simulink model "SMC_ThreeLayerApproach5TrackingNew"  (R2019b)
settings: Solver=FixedStepAuto  StartTime=0.0  StopTime=10.0  FixedStep=0.002  RelTol=1e-3
libraries: robotcorelib x1
settings Model: Creator=USER  LastModifiedBy=USER

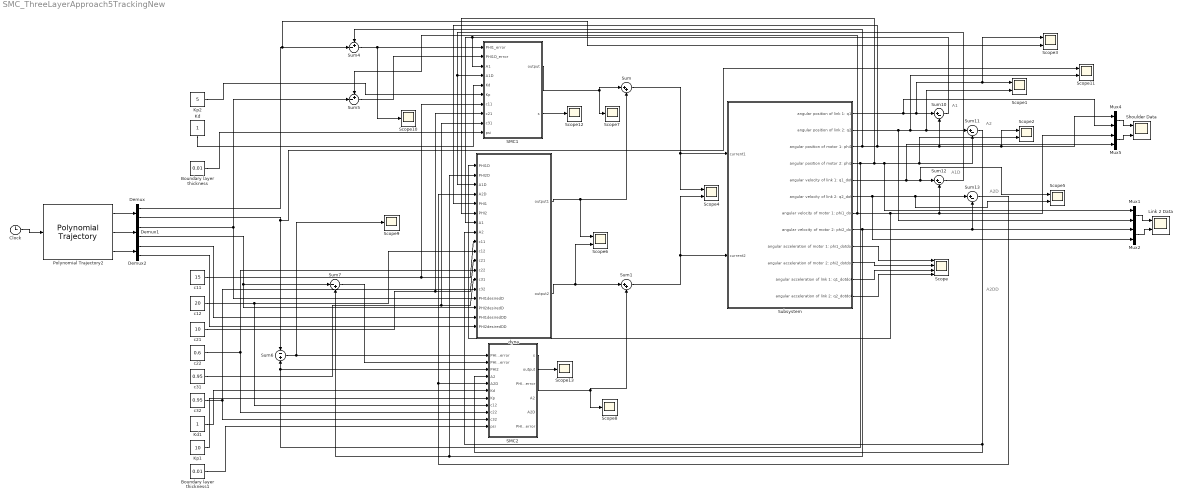
== system SMC_ThreeLayerApproach5TrackingNew ==
  note: A2D
  note: A2
  note: A1
  note: A1D
  note: A2DD
  Boundary layer thickness : Constant  Value=0.01
  Boundary layer thickness1 : Constant  Value=0.01  VectorParams1D=off
  Clock : Clock
  Demux : Demux  Outputs=2
  Demux1 : Demux  Outputs=2
  Demux2 : Demux  Outputs=2
  Kd : Constant
  Kd1 : Constant
  Kp1 : Constant  Value=10
  Kp2 : Constant  Value=5
  Link 2 Data : Scope  NumInputPorts=2
  Mux{1..2,4..5} (4 alike) : Mux  Inputs=2
  Polynomial Trajectory2 : robotcorelib/Polynomial Trajectory  WaypointSource=Internal  Waypoints=[ 0, pi/2; 0, pi/4 ]  TimePoints=[0,5]  TimeInterval=[ 1, 4 ]  Method=Cubic Polynomial  ParameterSource=Internal  VelocityBoundaryCondition=zeros( 2, 2 )  AccelerationBoundaryCondition=zeros( 2, 5 )  SimulateUsing=Interpreted execution
      settings: SourceProductName=Robotics System Toolbox  SourceProductBaseCode=RO
  SMC1 : MATLAB Function  TreatAsAtomicUnit=on
  SMC2 : MATLAB Function  TreatAsAtomicUnit=on
  Scope : Scope  NumInputPorts=4
  Scope{1..6,11} (7 alike) : Scope  NumInputPorts=2
  Scope{7..10,12..13} (6 alike) : Scope
  Shoulder Data : Scope  NumInputPorts=2
  Subsystem : Subsystem
  Sum : Sum  Inputs=|++
  Sum1 : Sum  Inputs=|++
  Sum{10..13} (4 alike) : Sum  Inputs=|+-
  Sum4 : Sum  Inputs=+-|
  Sum5 : Sum  Inputs=+-|
  Sum6 : Sum  Inputs=-|+
  Sum7 : Sum  Inputs=|-+
  c11 : Constant  Value=15
  c12 : Constant  Value=20
  c21 : Constant  Value=10
  c22 : Constant  Value=0.6
  c31 : Constant  Value=0.95
  c32 : Constant  Value=0.95
  dyna : MATLAB Function  TreatAsAtomicUnit=on
  wires:
  Mux2/1 -> Link 2 Data/2
  Kp1/1 -> SMC2/7(Kp)
  Sum7/1 -> SMC2/2("PHI2D_error ")
  Subsystem/12(angular acceleration of link 2: q2_dotdot) -> Scope/4
  Demux1/2 -> dyna/16(PHI2desiredD), Sum7/1
  Sum/1 -> Scope4/1, Subsystem/1(current1)
  Subsystem/10(angular acceleration of motor 2: phi2_dotdot) -> Scope/2
  Sum5/1 -> SMC1/2(PHI1D_error)
  c32/1 -> SMC2/10(c32), dyna/14(c32)
  Subsystem/9(angular acceleration of motor 1: phi1_dotdot) -> Scope/1
  Subsystem/8(angular velocity of motor 2: phi2_dot) -> dyna/2(PHI2D), Sum7/2, Mux2/1, Sum13/2
  dyna/1(output1) -> Scope6/1, Sum/2
  Subsystem/11(angular acceleration of link 1: q1_dotdot) -> Scope/3
  SMC1/1(output) -> Sum/1, Scope7/1
  c21/1 -> SMC1/8(c21), dyna/11(c21)
  Subsystem/6(angular velocity of link 2: q2_dot) -> Mux2/2, Scope5/2, Sum13/1
  Sum10/1 -> dyna/7(A1), SMC1/3(A1)
  Subsystem/4(angular position of motor 2: phi2) -> dyna/6(PHI2), Mux1/1, Scope2/2, Sum11/2, SMC2/3(PHI2), Sum6/2
  c31/1 -> SMC1/9(c31), dyna/13(c31)
  Sum12/1 -> SMC1/4(A1D), dyna/3(A1D)
  Sum11/1 -> SMC2/4("A2 "), dyna/8(A2)
  Kd/1 -> SMC1/5(Kd)
  Subsystem/2(angular position of link 2: q2) -> Mux1/2, Scope11/2, Scope1/2, Sum11/1
  Kd1/1 -> SMC2/6(Kd)
  Boundary layer thickness1/1 -> SMC2/11(psi)
  SMC2/2(output) -> Sum1/2, Scope8/1
  Subsystem/5(angular velocity of link 1: q1_dot) -> Mux5/2, Scope5/1, Sum12/1
  c11/1 -> SMC1/7(c11), dyna/9(c11)
  Sum4/1 -> Scope10/1, SMC1/1(PHI1_error)
  Subsystem/1(angular position of link 1: q1) -> Mux4/2, Scope3/1, Scope1/1, Sum10/1
  Mux4/1 -> Shoulder Data/1
  dyna/2(output2) -> Scope6/2, Sum1/1
  Sum6/1 -> Scope9/1, SMC2/1("PHI2_error ")
  Subsystem/7(angular velocity of motor 1: phi1_dot) -> dyna/1(PHI1D), Mux5/1, Sum12/2, Sum5/1
  Mux5/1 -> Shoulder Data/2
  Subsystem/3(angular position of motor 1: phi1) -> dyna/5(PHI1), Mux4/1, Scope2/1, Sum10/2, Sum4/1
  Sum13/1 -> dyna/4(A2D), SMC2/5("A2D ")
  Demux/2 -> Scope11/1, Sum6/1
  Sum1/1 -> Subsystem/2("current2 "), Scope4/2
  Demux/1 -> Scope3/2, Sum4/2
  Mux1/1 -> Link 2 Data/1
  c22/1 -> SMC2/9(c22), dyna/12(c22)
  Boundary layer thickness/1 -> SMC1/10(psi)
  Clock/1 -> Polynomial Trajectory2/1
  Kp2/1 -> SMC1/6(Kp)
  c12/1 -> SMC2/8(c12), dyna/10(c12)
  Polynomial Trajectory2/1 -> Demux/1
  Polynomial Trajectory2/2 -> Demux1/1
  Polynomial Trajectory2/3 -> Demux2/1
  Demux1/1 -> Sum5/2, dyna/15(PHI1desiredD)
  Demux2/1 -> dyna/17(PHI1desiredDD)
  Demux2/2 -> dyna/18(PHI2desiredDD)
  SMC1/2(s) -> Scope12/1
  SMC2/1(s) -> Scope13/1

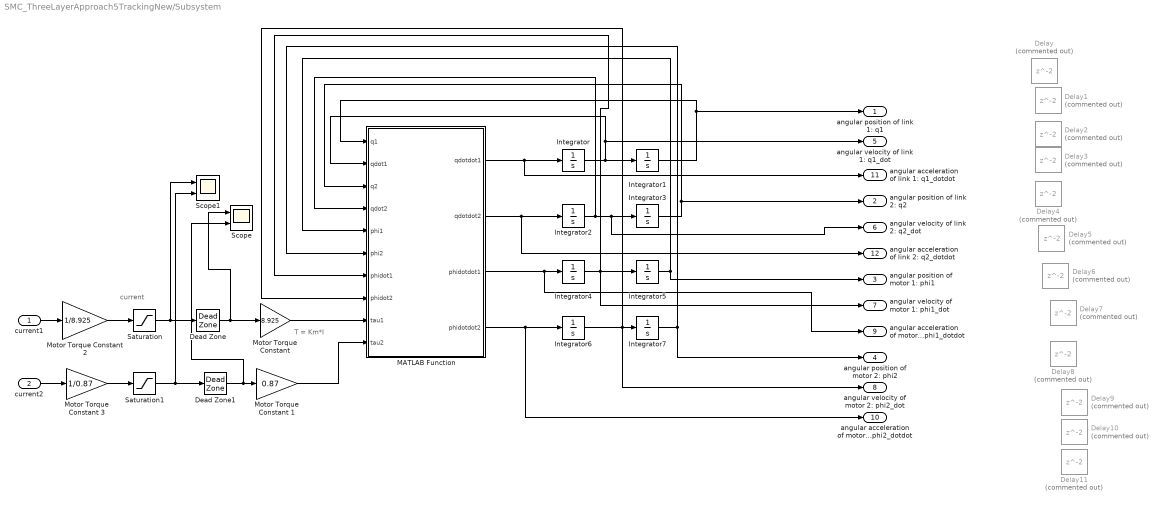
== system SMC_ThreeLayerApproach5TrackingNew/Subsystem ==
  note: current
  note: T = Km*I
  current1 : Inport
  "current2 " : Inport  Port=2
  Dead Zone : DeadZone  LowerValue=-0.165  UpperValue=0.183  ZeroCross=off  SaturateOnIntegerOverflow=on
  Dead Zone1 : DeadZone  LowerValue=-0.165  UpperValue=0.183  ZeroCross=off  SaturateOnIntegerOverflow=on
  Delay{,1..11} (12 alike) : Delay  Commented=on  SampleTime=0.002
  Integrator{,1..7} (8 alike) : Integrator
  MATLAB Function : MATLAB Function  TreatAsAtomicUnit=on
  "Motor Torque Constant " : Gain  Gain=8.925
  Motor Torque Constant 1 : Gain  Gain=0.87
  Motor Torque Constant 2 : Gain  Gain=1/8.925
  Motor Torque Constant 3 : Gain  Gain=1/0.87
  Saturation : Saturate  UpperLimit=0.94  LowerLimit=-0.94  ZeroCross=off
  Saturation1 : Saturate  UpperLimit=0.94  LowerLimit=-0.94  ZeroCross=off
  Scope : Scope  NumInputPorts=2
  Scope1 : Scope  NumInputPorts=2
  angular position of link 1: q1 : Outport
  angular position of link 2: q2 : Outport  Port=2
  angular position of motor 1: phi1 : Outport  Port=3
  angular position of motor 2: phi2 : Outport  Port=4
  angular velocity of link 1: q1_dot : Outport  Port=5
  angular velocity of link 2: q2_dot : Outport  Port=6
  angular velocity of motor 1: phi1_dot : Outport  Port=7
  angular velocity of motor 2: phi2_dot : Outport  Port=8
  angular acceleration of motor 1: phi1_dotdot : Outport  Port=9
  angular acceleration of motor 2: phi2_dotdot : Outport  Port=10
  angular acceleration of link 1: q1_dotdot : Outport  Port=11
  angular acceleration of link 2: q2_dotdot : Outport  Port=12
  wires:
  Saturation/1 -> Scope1/1, Dead Zone/1
  "Motor Torque Constant "/1 -> MATLAB Function/9(tau1)
  Motor Torque Constant 1/1 -> MATLAB Function/10(tau2)
  Dead Zone/1 -> Scope/1, "Motor Torque Constant "/1
  Dead Zone1/1 -> Scope/2, Motor Torque Constant 1/1
  current1/1 -> Motor Torque Constant 2/1
  "current2 "/1 -> Motor Torque Constant 3/1
  Motor Torque Constant 2/1 -> Saturation/1
  Motor Torque Constant 3/1 -> Saturation1/1
  Saturation1/1 -> Scope1/2, Dead Zone1/1
  Integrator1/1 -> angular position of link 1: q1/1, MATLAB Function/1(q1)
  Integrator/1 -> angular velocity of link 1: q1_dot/1, MATLAB Function/2(qdot1), Integrator1/1
  MATLAB Function/1(qdotdot1) -> angular acceleration of link 1: q1_dotdot/1, Integrator/1
  Integrator3/1 -> angular position of link 2: q2/1, MATLAB Function/3(q2)
  Integrator2/1 -> angular velocity of link 2: q2_dot/1, Integrator3/1, MATLAB Function/4(qdot2)
  MATLAB Function/2(qdotdot2) -> angular acceleration of link 2: q2_dotdot/1, Integrator2/1
  Integrator5/1 -> angular position of motor 1: phi1/1, MATLAB Function/5(phi1)
  MATLAB Function/3(phidotdot1) -> angular acceleration of motor 1: phi1_dotdot/1, Integrator4/1
  Integrator4/1 -> angular velocity of motor 1: phi1_dot/1, Integrator5/1, MATLAB Function/7(phidot1)
  Integrator6/1 -> angular velocity of motor 2: phi2_dot/1, MATLAB Function/8(phidot2), Integrator7/1
  MATLAB Function/4(phidotdot2) -> angular acceleration of motor 2: phi2_dotdot/1, Integrator6/1
  Integrator7/1 -> angular position of motor 2: phi2/1, MATLAB Function/6(phi2)

== matlab function SMC_ThreeLayerApproach5TrackingNew/dyna ==
  data: output1 output; PHI1D input; PHI2D input; A1D input; A2D input; output2 output; PHI1 input; PHI2 input; A1 input; A2 input; c11 input; c12 input; c21 input; c22 input; c31 input; c32 input; PHI1desiredD input; PHI2desiredD input; PHI1desiredDD input; PHI2desiredDD input
function [output1, output2]= dyna(PHI1D, PHI2D,A1D, A2D, PHI1, PHI2, A1, A2, c11, c12, c21, c22, c31, c32, PHI1desiredD, PHI2desiredD,PHI1desiredDD,PHI2desiredDD)
%Electrical School values
L1 = 0.343;
L2 = 0.267;
Lc1 = 0.1590;
Lc2 = 0.0550;
m1 = 1.51;
m2 = 0.87326;
I1 = 0.0392;
I2 = 0.0081;
B1 = 0.070364;
B2 = 0.028211;
Bm1 =4.5;
Bm2 = 0.5;
Ks1 = 9;
Ks2 = 4;
Ir1 = 0.0628;
Ir2 = 0.0026;
    
A1desiredD = 0;
A2desiredD = 0;
% PHI1desiredD = 0;
% PHI2desiredD = 0;
A1desiredDD = 0;
A2desiredDD = 0;
% PHI1desiredDD = 0;
% PHI2desiredDD = 0;

%derived from SMC_threeLayer.mlx
output1 = (c21*(A1D - A1desiredD) - PHI1desiredDD + c11*(PHI1D - PHI1desiredD) - c31*(A1desiredDD - (2*A2*I2^2*Ir1*Ks2 - 2*A1*I1^2*I2*Ks1 - 2*A1*I2^2*Ir1*Ks1 - 2*A1*I1*I2^2*Ks1 - A1*Ks1*L1^2*Lc2^4*m2^3 - A1*Ks1*L1^4*Lc2^2*m2^3 - 2*A1*I2^2*Ks1*L1^2*m2 - 2*A1*I2*Ks1*L1^4*m2^2 - 2*A1*I2^2*Ks1*Lc1^2*m1 - 2*A1*I1^2*Ks1*Lc2^2*m2 - 2*A1*I2*Ks1*Lc1^4*m1^2 - 2*A1*I1*Ks1*Lc2^4*m2^2 - 2*A1*Ir1*Ks1*Lc2^4*m2^2 + 2*A2*Ir1*Ks2*Lc2^4*m2^2 - 2*A1*I1*I2*Ir1*Ks1 + 2*A2*I1*I2*Ir1*Ks2 + A1*Ks1*L1^2*Lc2^4*m2^3*cos(2*A2 + 2*PHI2) + A1*Ks1*L1^4*Lc2^2*m2^3*cos(2*A2 + 2*PHI2) + A1*Ks1*L1^3*Lc2^3*m2^3*cos(3*A2 + 3*PHI2) - 3*A1*I1*Ks1*L1^2*Lc2^2*m2^2 - 3*A1*I2*Ks1*L1^2*Lc2^2*m2^2 - 2*A1*Ir1*Ks1*L1^2*Lc2^2*m2^2 + 4*A2*Ir1*Ks2*L1^2*Lc2^2*m2^2 - A1*Ks1*L1^3*Lc2^3*m2^3*cos(A2 + PHI2) + 2*A1D^2*Ir1*L1*Lc2^5*m2^3*sin(A2 + PHI2) + 2*A2D^2*Ir1*L1*Lc2^5*m2^3*sin(A2 + PHI2) - 2*A1*Ks1*Lc1^2*Lc2^4*m1*m2^2 - 2*A1*Ks1*Lc1^4*Lc2^2*m1^2*m2 + 2*Ir1*L1*Lc2^5*PHI1D^2*m2^3*sin(A2 + PHI2) + 2*Ir1*L1*Lc2^5*PHI2D^2*m2^3*sin(A2 + PHI2) + 3*A1D^2*Ir1*L1^2*Lc2^4*m2^3*sin(2*A2 + 2*PHI2) + A1D^2*Ir1*L1^4*Lc2^2*m2^3*sin(2*A2 + 2*PHI2) + 2*A2D^2*Ir1*L1^2*Lc2^4*m2^3*sin(2*A2 + 2*PHI2) + A1D^2*Ir1*L1^3*Lc2^3*m2^3*sin(3*A2 + 3*PHI2) - 4*A1*I1*I2*Ks1*L1^2*m2 - 4*A1*I1*I2*Ks1*Lc1^2*m1 - 4*A1*I1*I2*Ks1*Lc2^2*m2 - 2*A1*I2*Ir1*Ks1*L1^2*m2 + 2*A2*I2*Ir1*Ks2*L1^2*m2 - 2*A1*I2*Ir1*Ks1*Lc1^2*m1 - 2*A1*I1*Ir1*Ks1*Lc2^2*m2 - 4*A1*I2*Ir1*Ks1*Lc2^2*m2 + 2*A2*I2*Ir1*Ks2*Lc1^2*m1 + 2*A2*I1*Ir1*Ks2*Lc2^2*m2 + 4*A2*I2*Ir1*Ks2*Lc2^2*m2 + 3*Ir1*L1^2*Lc2^4*PHI1D^2*m2^3*sin(2*A2 + 2*PHI2) + Ir1*L1^4*Lc2^2*PHI1D^2*m2^3*sin(2*A2 + 2*PHI2) + 2*Ir1*L1^2*Lc2^4*PHI2D^2*m2^3*sin(2*A2 + 2*PHI2) + Ir1*L1^3*Lc2^3*PHI1D^2*m2^3*sin(3*A2 + 3*PHI2) + 3*A1D^2*Ir1*L1^3*Lc2^3*m2^3*sin(A2 + PHI2) + 2*A2D^2*Ir1*L1^3*Lc2^3*m2^3*sin(A2 + PHI2) + 3*Ir1*L1^3*Lc2^3*PHI1D^2*m2^3*sin(A2 + PHI2) + 2*Ir1*L1^3*Lc2^3*PHI2D^2*m2^3*sin(A2 + PHI2) - 3*A1*Ks1*L1^2*Lc1^2*Lc2^2*m1*m2^2 - 4*A1*I1*Ks1*L1*Lc2^3*m2^2*cos(A2 + PHI2) - 4*A1*I2*Ks1*L1^3*Lc2*m2^2*cos(A2 + PHI2) - 4*A1*Ir1*Ks1*L1*Lc2^3*m2^2*cos(A2 + PHI2) + 6*A2*Ir1*Ks2*L1*Lc2^3*m2^2*cos(A2 + PHI2) + 2*A2*Ir1*Ks2*L1^3*Lc2*m2^2*cos(A2 + PHI2) + 4*A1D*A2D*Ir1*L1*Lc2^5*m2^3*sin(A2 + PHI2) + 2*A1D^2*I2^2*Ir1*L1*Lc2*m2*sin(A2 + PHI2) + 2*A2D^2*I2^2*Ir1*L1*Lc2*m2*sin(A2 + PHI2) + 4*A1D*Ir1*L1*Lc2^5*PHI1D*m2^3*sin(A2 + PHI2) + 4*A1D*Ir1*L1*Lc2^5*PHI2D*m2^3*sin(A2 + PHI2) + 4*A2D*Ir1*L1*Lc2^5*PHI1D*m2^3*sin(A2 + PHI2) + 4*A2D*Ir1*L1*Lc2^5*PHI2D*m2^3*sin(A2 + PHI2) - 4*A1*I2*Ks1*L1^2*Lc1^2*m1*m2 - 4*A1*I1*Ks1*Lc1^2*Lc2^2*m1*m2 - 4*A1*I2*Ks1*Lc1^2*Lc2^2*m1*m2 - 2*A1*Ir1*Ks1*Lc1^2*Lc2^2*m1*m2 + 2*A2*Ir1*Ks2*Lc1^2*Lc2^2*m1*m2 + 2*I2^2*Ir1*L1*Lc2*PHI1D^2*m2*sin(A2 + PHI2) + 2*I2^2*Ir1*L1*Lc2*PHI2D^2*m2*sin(A2 + PHI2) + A1*I1*Ks1*L1^2*Lc2^2*m2^2*cos(2*A2 + 2*PHI2) + A1*I2*Ks1*L1^2*Lc2^2*m2^2*cos(2*A2 + 2*PHI2) + 2*A2*Ir1*Ks2*L1^2*Lc2^2*m2^2*cos(2*A2 + 2*PHI2) + 4*A1D*A2D*Ir1*L1^2*Lc2^4*m2^3*sin(2*A2 + 2*PHI2) + 4*Ir1*L1*Lc2^5*PHI1D*PHI2D*m2^3*sin(A2 + PHI2) + 6*A1D*Ir1*L1^2*Lc2^4*PHI1D*m2^3*sin(2*A2 + 2*PHI2) + 2*A1D*Ir1*L1^4*Lc2^2*PHI1D*m2^3*sin(2*A2 + 2*PHI2) + 4*A1D*Ir1*L1^2*Lc2^4*PHI2D*m2^3*sin(2*A2 + 2*PHI2) + 4*A2D*Ir1*L1^2*Lc2^4*PHI1D*m2^3*sin(2*A2 + 2*PHI2) + 2*A1D*Ir1*L1^3*Lc2^3*PHI1D*m2^3*sin(3*A2 + 3*PHI2) + 4*A2D*Ir1*L1^2*Lc2^4*PHI2D*m2^3*sin(2*A2 + 2*PHI2) + 4*Ir1*L1^2*Lc2^4*PHI1D*PHI2D*m2^3*sin(2*A2 + 2*PHI2) + 4*A1D*A2D*Ir1*L1^3*Lc2^3*m2^3*sin(A2 + PHI2) + 2*A1D^2*I1*Ir1*L1*Lc2^3*m2^2*sin(A2 + PHI2) + 4*A1D^2*I2*Ir1*L1*Lc2^3*m2^2*sin(A2 + PHI2) + 2*A1D^2*I2*Ir1*L1^3*Lc2*m2^2*sin(A2 + PHI2) + 2*A2D^2*I1*Ir1*L1*Lc2^3*m2^2*sin(A2 + PHI2) + 4*A2D^2*I2*Ir1*L1*Lc2^3*m2^2*sin(A2 + PHI2) + 2*A2D^2*I2*Ir1*L1^3*Lc2*m2^2*sin(A2 + PHI2) + 6*A1D*Ir1*L1^3*Lc2^3*PHI1D*m2^3*sin(A2 + PHI2) + 4*A1D*Ir1*L1^3*Lc2^3*PHI2D*m2^3*sin(A2 + PHI2) + 4*A2D*Ir1*L1^3*Lc2^3*PHI1D*m2^3*sin(A2 + PHI2) + 4*A2D*Ir1*L1^3*Lc2^3*PHI2D*m2^3*sin(A2 + PHI2) + 2*I1*Ir1*L1*Lc2^3*PHI1D^2*m2^2*sin(A2 + PHI2) + 2*I1*Ir1*L1*Lc2^3*PHI2D^2*m2^2*sin(A2 + PHI2) + 4*I2*Ir1*L1*Lc2^3*PHI1D^2*m2^2*sin(A2 + PHI2) + 2*I2*Ir1*L1^3*Lc2*PHI1D^2*m2^2*sin(A2 + PHI2) + 4*I2*Ir1*L1*Lc2^3*PHI2D^2*m2^2*sin(A2 + PHI2) + 2*I2*Ir1*L1^3*Lc2*PHI2D^2*m2^2*sin(A2 + PHI2) + 4*Ir1*L1^3*Lc2^3*PHI1D*PHI2D*m2^3*sin(A2 + PHI2) + A1D^2*I1*Ir1*L1^2*Lc2^2*m2^2*sin(2*A2 + 2*PHI2) + 3*A1D^2*I2*Ir1*L1^2*Lc2^2*m2^2*sin(2*A2 + 2*PHI2) + 2*A2D^2*I2*Ir1*L1^2*Lc2^2*m2^2*sin(2*A2 + 2*PHI2) + I1*Ir1*L1^2*Lc2^2*PHI1D^2*m2^2*sin(2*A2 + 2*PHI2) + 3*I2*Ir1*L1^2*Lc2^2*PHI1D^2*m2^2*sin(2*A2 + 2*PHI2) + 2*I2*Ir1*L1^2*Lc2^2*PHI2D^2*m2^2*sin(2*A2 + 2*PHI2) - 4*A1*Ks1*L1*Lc1^2*Lc2^3*m1*m2^2*cos(A2 + PHI2) + A1*Ks1*L1^2*Lc1^2*Lc2^2*m1*m2^2*cos(2*A2 + 2*PHI2) + 4*A1D*A2D*I2^2*Ir1*L1*Lc2*m2*sin(A2 + PHI2) + 2*A1D^2*I1*I2*Ir1*L1*Lc2*m2*sin(A2 + PHI2) + 2*A2D^2*I1*I2*Ir1*L1*Lc2*m2*sin(A2 + PHI2) + 4*A1D*I2^2*Ir1*L1*Lc2*PHI1D*m2*sin(A2 + PHI2) + 4*A1D*I2^2*Ir1*L1*Lc2*PHI2D*m2*sin(A2 + PHI2) + 4*A2D*I2^2*Ir1*L1*Lc2*PHI1D*m2*sin(A2 + PHI2) + 4*A2D*I2^2*Ir1*L1*Lc2*PHI2D*m2*sin(A2 + PHI2) + 2*I1*I2*Ir1*L1*Lc2*PHI1D^2*m2*sin(A2 + PHI2) + 2*I1*I2*Ir1*L1*Lc2*PHI2D^2*m2*sin(A2 + PHI2) + 4*I2^2*Ir1*L1*Lc2*PHI1D*PHI2D*m2*sin(A2 + PHI2) + 2*A1D^2*Ir1*L1*Lc1^2*Lc2^3*m1*m2^2*sin(A2 + PHI2) + 2*A2D^2*Ir1*L1*Lc1^2*Lc2^3*m1*m2^2*sin(A2 + PHI2) + 2*Ir1*L1*Lc1^2*Lc2^3*PHI1D^2*m1*m2^2*sin(A2 + PHI2) + 2*Ir1*L1*Lc1^2*Lc2^3*PHI2D^2*m1*m2^2*sin(A2 + PHI2) + 4*A1D*A2D*I1*Ir1*L1*Lc2^3*m2^2*sin(A2 + PHI2) + 8*A1D*A2D*I2*Ir1*L1*Lc2^3*m2^2*sin(A2 + PHI2) + 4*A1D*A2D*I2*Ir1*L1^3*Lc2*m2^2*sin(A2 + PHI2) + A1D^2*Ir1*L1^2*Lc1^2*Lc2^2*m1*m2^2*sin(2*A2 + 2*PHI2) + 4*A1D*I1*Ir1*L1*Lc2^3*PHI1D*m2^2*sin(A2 + PHI2) + 4*A1D*I1*Ir1*L1*Lc2^3*PHI2D*m2^2*sin(A2 + PHI2) + 8*A1D*I2*Ir1*L1*Lc2^3*PHI1D*m2^2*sin(A2 + PHI2) + 4*A1D*I2*Ir1*L1^3*Lc2*PHI1D*m2^2*sin(A2 + PHI2) + 4*A2D*I1*Ir1*L1*Lc2^3*PHI1D*m2^2*sin(A2 + PHI2) + 8*A1D*I2*Ir1*L1*Lc2^3*PHI2D*m2^2*sin(A2 + PHI2) + 4*A1D*I2*Ir1*L1^3*Lc2*PHI2D*m2^2*sin(A2 + PHI2) + 4*A2D*I1*Ir1*L1*Lc2^3*PHI2D*m2^2*sin(A2 + PHI2) + 8*A2D*I2*Ir1*L1*Lc2^3*PHI1D*m2^2*sin(A2 + PHI2) + 4*A2D*I2*Ir1*L1^3*Lc2*PHI1D*m2^2*sin(A2 + PHI2) + 8*A2D*I2*Ir1*L1*Lc2^3*PHI2D*m2^2*sin(A2 + PHI2) + 4*A2D*I2*Ir1*L1^3*Lc2*PHI2D*m2^2*sin(A2 + PHI2) + Ir1*L1^2*Lc1^2*Lc2^2*PHI1D^2*m1*m2^2*sin(2*A2 + 2*PHI2) + 4*A1D*A2D*I2*Ir1*L1^2*Lc2^2*m2^2*sin(2*A2 + 2*PHI2) + 4*I1*Ir1*L1*Lc2^3*PHI1D*PHI2D*m2^2*sin(A2 + PHI2) + 8*I2*Ir1*L1*Lc2^3*PHI1D*PHI2D*m2^2*sin(A2 + PHI2) + 4*I2*Ir1*L1^3*Lc2*PHI1D*PHI2D*m2^2*sin(A2 + PHI2) + 2*A1D*I1*Ir1*L1^2*Lc2^2*PHI1D*m2^2*sin(2*A2 + 2*PHI2) + 6*A1D*I2*Ir1*L1^2*Lc2^2*PHI1D*m2^2*sin(2*A2 + 2*PHI2) + 4*A1D*I2*Ir1*L1^2*Lc2^2*PHI2D*m2^2*sin(2*A2 + 2*PHI2) + 4*A2D*I2*Ir1*L1^2*Lc2^2*PHI1D*m2^2*sin(2*A2 + 2*PHI2) + 4*A2D*I2*Ir1*L1^2*Lc2^2*PHI2D*m2^2*sin(2*A2 + 2*PHI2) - 4*A1*I1*I2*Ks1*L1*Lc2*m2*cos(A2 + PHI2) - 4*A1*I2*Ir1*Ks1*L1*Lc2*m2*cos(A2 + PHI2) + 2*A2*I1*Ir1*Ks2*L1*Lc2*m2*cos(A2 + PHI2) + 6*A2*I2*Ir1*Ks2*L1*Lc2*m2*cos(A2 + PHI2) + 4*I2*Ir1*L1^2*Lc2^2*PHI1D*PHI2D*m2^2*sin(2*A2 + 2*PHI2) + 2*A1D^2*I2*Ir1*L1*Lc1^2*Lc2*m1*m2*sin(A2 + PHI2) + 2*A2D^2*I2*Ir1*L1*Lc1^2*Lc2*m1*m2*sin(A2 + PHI2) + 2*I2*Ir1*L1*Lc1^2*Lc2*PHI1D^2*m1*m2*sin(A2 + PHI2) + 2*I2*Ir1*L1*Lc1^2*Lc2*PHI2D^2*m1*m2*sin(A2 + PHI2) + 4*A1D*A2D*I1*I2*Ir1*L1*Lc2*m2*sin(A2 + PHI2) + 4*A1D*I1*I2*Ir1*L1*Lc2*PHI1D*m2*sin(A2 + PHI2) + 4*A1D*I1*I2*Ir1*L1*Lc2*PHI2D*m2*sin(A2 + PHI2) + 4*A2D*I1*I2*Ir1*L1*Lc2*PHI1D*m2*sin(A2 + PHI2) + 4*A2D*I1*I2*Ir1*L1*Lc2*PHI2D*m2*sin(A2 + PHI2) + 4*I1*I2*Ir1*L1*Lc2*PHI1D*PHI2D*m2*sin(A2 + PHI2) + 4*A1D*A2D*Ir1*L1*Lc1^2*Lc2^3*m1*m2^2*sin(A2 + PHI2) + 4*A1D*Ir1*L1*Lc1^2*Lc2^3*PHI1D*m1*m2^2*sin(A2 + PHI2) + 4*A1D*Ir1*L1*Lc1^2*Lc2^3*PHI2D*m1*m2^2*sin(A2 + PHI2) + 4*A2D*Ir1*L1*Lc1^2*Lc2^3*PHI1D*m1*m2^2*sin(A2 + PHI2) + 4*A2D*Ir1*L1*Lc1^2*Lc2^3*PHI2D*m1*m2^2*sin(A2 + PHI2) + 4*Ir1*L1*Lc1^2*Lc2^3*PHI1D*PHI2D*m1*m2^2*sin(A2 + PHI2) + 2*A1D*Ir1*L1^2*Lc1^2*Lc2^2*PHI1D*m1*m2^2*sin(2*A2 + 2*PHI2) - 4*A1*I2*Ks1*L1*Lc1^2*Lc2*m1*m2*cos(A2 + PHI2) + 2*A2*Ir1*Ks2*L1*Lc1^2*Lc2*m1*m2*cos(A2 + PHI2) + 4*A1D*I2*Ir1*L1*Lc1^2*Lc2*PHI1D*m1*m2*sin(A2 + PHI2) + 4*A1D*I2*Ir1*L1*Lc1^2*Lc2*PHI2D*m1*m2*sin(A2 + PHI2) + 4*A2D*I2*Ir1*L1*Lc1^2*Lc2*PHI1D*m1*m2*sin(A2 + PHI2) + 4*A2D*I2*Ir1*L1*Lc1^2*Lc2*PHI2D*m1*m2*sin(A2 + PHI2) + 4*I2*Ir1*L1*Lc1^2*Lc2*PHI1D*PHI2D*m1*m2*sin(A2 + PHI2) + 4*A1D*A2D*I2*Ir1*L1*Lc1^2*Lc2*m1*m2*sin(A2 + PHI2))/(Ir1*(2*I1*I2^2 + 2*I1^2*I2 + 2*I2^2*L1^2*m2 + 2*I2*L1^4*m2^2 + 2*I2^2*Lc1^2*m1 + 2*I1^2*Lc2^2*m2 + 2*I2*Lc1^4*m1^2 + 2*I1*Lc2^4*m2^2 + L1^2*Lc2^4*m2^3 + L1^4*Lc2^2*m2^3 + 4*I1*I2*L1^2*m2 + 4*I1*I2*Lc1^2*m1 + 4*I1*I2*Lc2^2*m2 - L1^2*Lc2^4*m2^3*cos(2*A2 + 2*PHI2) - L1^4*Lc2^2*m2^3*cos(2*A2 + 2*PHI2) - L1^3*Lc2^3*m2^3*cos(3*A2 + 3*PHI2) + 3*I1*L1^2*Lc2^2*m2^2 + 3*I2*L1^2*Lc2^2*m2^2 + L1^3*Lc2^3*m2^3*cos(A2 + PHI2) + 2*Lc1^2*Lc2^4*m1*m2^2 + 2*Lc1^4*Lc2^2*m1^2*m2 + 3*L1^2*Lc1^2*Lc2^2*m1*m2^2 + 4*I1*L1*Lc2^3*m2^2*cos(A2 + PHI2) + 4*I2*L1^3*Lc2*m2^2*cos(A2 + PHI2) + 4*I2*L1^2*Lc1^2*m1*m2 + 4*I1*Lc1^2*Lc2^2*m1*m2 + 4*I2*Lc1^2*Lc2^2*m1*m2 - I1*L1^2*Lc2^2*m2^2*cos(2*A2 + 2*PHI2) - I2*L1^2*Lc2^2*m2^2*cos(2*A2 + 2*PHI2) + 4*I1*I2*L1*Lc2*m2*cos(A2 + PHI2) + 4*L1*Lc1^2*Lc2^3*m1*m2^2*cos(A2 + PHI2) - L1^2*Lc1^2*Lc2^2*m1*m2^2*cos(2*A2 + 2*PHI2) + 4*I2*L1*Lc1^2*Lc2*m1*m2*cos(A2 + PHI2)))) + (A1*Ks1)/Ir1)/(c31/Ir1 - 1/Ir1);
output2 = -(c22*(A2D - A2desiredD) - PHI2desiredDD + c12*(PHI2D - PHI2desiredD) - c32*(A2desiredDD + (2*(A2*I1*I2*Ks2 - A1*I2*Ir2*Ks1 + A2*I1*Ir2*Ks2 + A2*I2*Ir2*Ks2 + (A2*Ks2*L1^2*Lc2^2*m2^2)/2 + A2*I2*Ks2*L1^2*m2 + A2*I2*Ks2*Lc1^2*m1 + A2*I1*Ks2*Lc2^2*m2 + A2*Ir2*Ks2*L1^2*m2 - A1*Ir2*Ks1*Lc2^2*m2 + A2*Ir2*Ks2*Lc1^2*m1 + A2*Ir2*Ks2*Lc2^2*m2 + A2*Ks2*Lc1^2*Lc2^2*m1*m2 - (A2*Ks2*L1^2*Lc2^2*m2^2*cos(2*A2 + 2*PHI2))/2 + A1D^2*Ir2*L1*Lc2^3*m2^2*sin(A2 + PHI2) + A1D^2*Ir2*L1^3*Lc2*m2^2*sin(A2 + PHI2) + A2D^2*Ir2*L1*Lc2^3*m2^2*sin(A2 + PHI2) + Ir2*L1*Lc2^3*PHI1D^2*m2^2*sin(A2 + PHI2) + Ir2*L1^3*Lc2*PHI1D^2*m2^2*sin(A2 + PHI2) + Ir2*L1*Lc2^3*PHI2D^2*m2^2*sin(A2 + PHI2) + A1D^2*Ir2*L1^2*Lc2^2*m2^2*sin(2*A2 + 2*PHI2) + (A2D^2*Ir2*L1^2*Lc2^2*m2^2*sin(2*A2 + 2*PHI2))/2 + Ir2*L1^2*Lc2^2*PHI1D^2*m2^2*sin(2*A2 + 2*PHI2) + (Ir2*L1^2*Lc2^2*PHI2D^2*m2^2*sin(2*A2 + 2*PHI2))/2 + I1*Ir2*L1*Lc2*PHI1D^2*m2*sin(A2 + PHI2) + I2*Ir2*L1*Lc2*PHI1D^2*m2*sin(A2 + PHI2) + I2*Ir2*L1*Lc2*PHI2D^2*m2*sin(A2 + PHI2) + 2*A1D*A2D*Ir2*L1*Lc2^3*m2^2*sin(A2 + PHI2) + 2*A1D*Ir2*L1*Lc2^3*PHI1D*m2^2*sin(A2 + PHI2) + 2*A1D*Ir2*L1^3*Lc2*PHI1D*m2^2*sin(A2 + PHI2) + 2*A1D*Ir2*L1*Lc2^3*PHI2D*m2^2*sin(A2 + PHI2) + 2*A2D*Ir2*L1*Lc2^3*PHI1D*m2^2*sin(A2 + PHI2) + 2*A2D*Ir2*L1*Lc2^3*PHI2D*m2^2*sin(A2 + PHI2) + A1D*A2D*Ir2*L1^2*Lc2^2*m2^2*sin(2*A2 + 2*PHI2) + 2*Ir2*L1*Lc2^3*PHI1D*PHI2D*m2^2*sin(A2 + PHI2) + 2*A1D*Ir2*L1^2*Lc2^2*PHI1D*m2^2*sin(2*A2 + 2*PHI2) + A1D*Ir2*L1^2*Lc2^2*PHI2D*m2^2*sin(2*A2 + 2*PHI2) + A2D*Ir2*L1^2*Lc2^2*PHI1D*m2^2*sin(2*A2 + 2*PHI2) + A2D*Ir2*L1^2*Lc2^2*PHI2D*m2^2*sin(2*A2 + 2*PHI2) - A1*Ir2*Ks1*L1*Lc2*m2*cos(A2 + PHI2) + 2*A2*Ir2*Ks2*L1*Lc2*m2*cos(A2 + PHI2) + Ir2*L1^2*Lc2^2*PHI1D*PHI2D*m2^2*sin(2*A2 + 2*PHI2) + A1D^2*I1*Ir2*L1*Lc2*m2*sin(A2 + PHI2) + A1D^2*I2*Ir2*L1*Lc2*m2*sin(A2 + PHI2) + A2D^2*I2*Ir2*L1*Lc2*m2*sin(A2 + PHI2) + A1D^2*Ir2*L1*Lc1^2*Lc2*m1*m2*sin(A2 + PHI2) + Ir2*L1*Lc1^2*Lc2*PHI1D^2*m1*m2*sin(A2 + PHI2) + 2*A1D*A2D*I2*Ir2*L1*Lc2*m2*sin(A2 + PHI2) + 2*A1D*I1*Ir2*L1*Lc2*PHI1D*m2*sin(A2 + PHI2) + 2*A1D*I2*Ir2*L1*Lc2*PHI1D*m2*sin(A2 + PHI2) + 2*A1D*I2*Ir2*L1*Lc2*PHI2D*m2*sin(A2 + PHI2) + 2*A2D*I2*Ir2*L1*Lc2*PHI1D*m2*sin(A2 + PHI2) + 2*A2D*I2*Ir2*L1*Lc2*PHI2D*m2*sin(A2 + PHI2) + 2*I2*Ir2*L1*Lc2*PHI1D*PHI2D*m2*sin(A2 + PHI2) + 2*A1D*Ir2*L1*Lc1^2*Lc2*PHI1D*m1*m2*sin(A2 + PHI2)))/(Ir2*(2*I1*I2 + L1^2*Lc2^2*m2^2 + 2*I2*L1^2*m2 + 2*I2*Lc1^2*m1 + 2*I1*Lc2^2*m2 + 2*Lc1^2*Lc2^2*m1*m2 - L1^2*Lc2^2*m2^2*cos(2*A2 + 2*PHI2)))) + (A2*Ks2)/Ir2)/(1/Ir2 - (2*c32*(I1*I2 + (L1^2*Lc2^2*m2^2)/2 + I2*L1^2*m2 + I2*Lc1^2*m1 + I1*Lc2^2*m2 + Lc1^2*Lc2^2*m1*m2 - (L1^2*Lc2^2*m2^2*cos(2*A2 + 2*PHI2))/2))/(Ir2*(2*I1*I2 + L1^2*Lc2^2*m2^2 + 2*I2*L1^2*m2 + 2*I2*Lc1^2*m1 + 2*I1*Lc2^2*m2 + 2*Lc1^2*Lc2^2*m1*m2 - L1^2*Lc2^2*m2^2*cos(2*A2 + 2*PHI2))));

end

== matlab function SMC_ThreeLayerApproach5TrackingNew/Subsystem/MATLAB Function ==
  data: q1 input; qdotdot1 output; qdot1 input; q2 input; qdot2 input; phi1 input; phi2 input; phidot1 input; phidot2 input; tau1 input; tau2 input; qdotdot2 output; phidotdot1 output; phidotdot2 output
function [qdotdot1,qdotdot2,phidotdot1,phidotdot2] = fcn(q1,qdot1,q2,qdot2,phi1,phi2,phidot1,phidot2,tau1,tau2)
%y is thetadotdot
tau = [0;0;tau1;tau2];
%Veltman Thesis Values
% m1 = 0.5; 
% m2 = 1;
% L1 = 0.343;
% L2 = 0.267;
% Lc1 = 0.2;
% Lc2 = 0.25;
% I1 = 0.01;
% I2 = 0.01;
% B1 = 0.070364;
% B2 = 0.028211;

%Electrical School values
L1 = 0.343;
L2 = 0.267;
Lc1 = 0.1590;
Lc2 = 0.0550;
m1 = 1.51;
m2 = 0.87326;
I1 = 0.0392;
I2 = 0.0081;
B1 = 0.070364;
B2 = 0.028211;
Bm1 =4.5;
Bm2 = 0.5;
Ks1 = 9;
Ks2 = 4;
Ir1 = 0.0628;
Ir2 = 0.0026;

z = [0 0;
     0 0];
M11 = I2+I1+m2*((L1^2)+(Lc2^2)+2*L1*Lc2*cos(q2))+m1*(Lc1^2);
M12 = I2+m2*(Lc2^2)+L1*Lc2*m2*cos(q2);
M21 = M12;
M22 = I2+m2*(Lc2^2);

M1 = [M11 M12;
     M21 M22];

M2 = [Ir1 0;
      0 Ir2];
  
M = [M1 z;
     z  M2];
 
C11 = -m2*L1*Lc2*sin(q2)*qdot2;
C12 = -m2*L1*Lc2*sin(q2)*qdot2-m2*L1*Lc2*sin(q2)*qdot1;
C21 = m2*L1*Lc2*sin(q2)*qdot1;
C22 = 0;

Ca = [C11 C12;
     C21 C22];

C = [Ca z;
     z  z];
 
K1 = [Ks1 0;
      0  Ks2];
  
K = [K1 -K1;
     -K1 K1];
 
fvl = [B1 0;
      0  B2];
  
fvm = [Bm1 0;
       0  Bm2];
   
fv = [fvl z;
      z  fvm];
  
fvf = fv*[qdot1;qdot2;phidot1;phidot2];
Cf = C*[qdot1;qdot2;phidot1;phidot2];
Kf = K*[q1;q2;phi1;phi2];

y = inv(M)*(tau-Cf-fvf-Kf);
qdotdot1 = y(1);
qdotdot2 = y(2);
phidotdot1 = y(3);
phidotdot2 = y(4);

== matlab function SMC_ThreeLayerApproach5TrackingNew/SMC1 ==
  data: PHI1_error input; output output; PHI1D_error input; A1 input; A1D input; Kd input; Kp input; c11 input; c21 input; c31 input; psi input; s output
function [output,s] = smc(PHI1_error, PHI1D_error, A1, A1D, Kd, Kp, c11, c21, c31, psi)

    L1 = 0.343;
    L2 = 0.267;
    Lc1 = 0.1590;
    Lc2 = 0.0550;
    m1 = 1.51;
    m2 = 0.87326;
    I1 = 0.0392;
    I2 = 0.0081;
    B1 = 0.070364;
    B2 = 0.028211;
    Bm1 =4.5;
    Bm2 = 0.5;
    Ks1 = 9;
    Ks2 = 4;
    Ir1 = 0.0628;
    Ir2 = 0.0026;
    A1desired = 0;
    A1desiredD = 0;
    s = PHI1D_error + c21*(A1 - A1desired) + c31*(A1D - A1desiredD) + c11*(PHI1_error);

    if (abs(s) > psi)    
        sat_s = sign(s);
    else
        sat_s = s/psi;
    end
    
%     output = -Kd * sat_s - Kp*s;
    
    output = -Ir1*(-Kd * sat_s - Kp*s)/(c31-1);
end

== matlab function SMC_ThreeLayerApproach5TrackingNew/SMC2 ==
  data: s output; PHI2_error input; output output; PHI2D_error input; PHI2 input; A2 input; A2D input; Kd input; Kp input; c12 input; c22 input; c32 input; psi input; PHI2D_error output; A2 output; A2D output; PHI2_error output
function [s,output,PHI2D_error,A2,A2D,PHI2_error] = smc(PHI2_error, PHI2D_error,PHI2, A2,A2D, Kd, Kp, c12, c22, c32, psi)


    A2desired = 0;
    A2desiredD = 0;
    L1 = 0.343;
    L2 = 0.267;
    Lc1 = 0.1590;
    Lc2 = 0.0550;
    m1 = 1.51;
    m2 = 0.87326;
    I1 = 0.0392;
    I2 = 0.0081;
    B1 = 0.070364;
    B2 = 0.028211;
    Bm1 =4.5;
    Bm2 = 0.5;
    Ks1 = 9;
    Ks2 = 4;
    Ir1 = 0.0628;
    Ir2 = 0.0026;
    A1desired = 0;
    A1desiredD = 0;
    
    s = PHI2D_error + c22*(A2 - A2desired) + c32*(A2D - A2desiredD) + c12*(PHI2_error);
        
    if (abs(s) > psi)    
        sat_s = sign(s);
    else
        sat_s = s/psi;
    end
    
    output = (-Kd * sat_s - Kp*s)/(1/Ir2 - (2*c32*(I1*I2 + (L1^2*Lc2^2*m2^2)/2 + I2*L1^2*m2 + I2*Lc1^2*m1 + I1*Lc2^2*m2 + Lc1^2*Lc2^2*m1*m2 - (L1^2*Lc2^2*m2^2*cos(2*A2 + 2*PHI2))/2))/(Ir2*(2*I1*I2 + L1^2*Lc2^2*m2^2 + 2*I2*L1^2*m2 + 2*I2*Lc1^2*m1 + 2*I1*Lc2^2*m2 + 2*Lc1^2*Lc2^2*m1*m2 - L1^2*Lc2^2*m2^2*cos(2*A2 + 2*PHI2))));

end
